simulink model "SoC_modelbased"  (Simulink 10.2)
settings: Solver=ode45  StartTime=0.0  StopTime=75000  RelTol=1e-3  EnableMultiTasking=on
undefined symbols (not defined in the file or in its folder): battery_capacity, capacity_reduction_factor
libraries: pid_lib x1
settings Model: Creator=giovanni  LastModifiedBy=marcomussi
settings DataIOCC: LimitDataPoints=on
settings OptimizationCC: ExpressionDepthLimit=2147483647
settings DebuggingCC: AlgebraicLoopMsg=none  SolverPrmCheckMsg=warning  StateNameClashWarn=warning
settings ConfigComp: CovSFcnEnable=off

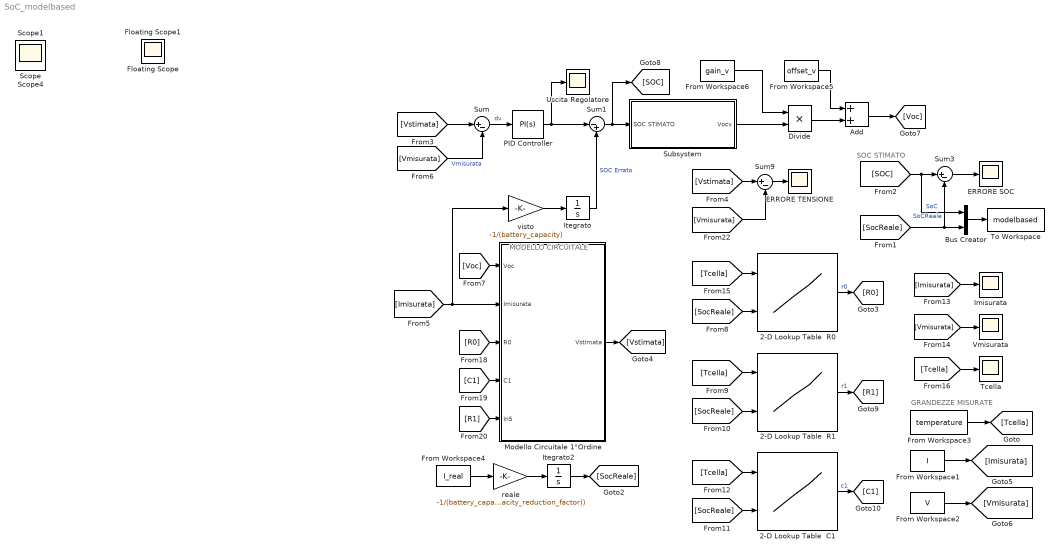
== system SoC_modelbased ==
  note: GRANDEZZE MISURATE
  note: MODELLO CIRCUITALE
  note: SOC STIMATO
  2-D Lookup Table  C1 : Lookup_n-D  BreakpointsForDimension1=[2 10 20 30 40]  BreakpointsForDimension2=|  Table=|  ExtrapMethod=Clip  UseLastTableValue=on  RndMeth=Simplest  InputSameDT=on
      BreakpointsForDimension2=|
      | [0.163145513075157	0.212319317933106	0.261240559284839	0.310166932050155	0.359120506846337	0.408117376969695	0.457142933463410	0.506212254204039	0.555338838203931	0.604575150487779	0.653951958006247	0.703454663475372	0.753095676425974	0.802798623734601	0.852544469586437	0.902318454030865	0.952029425469133
      | ]
      Table=|
      | reshape([4883.03519070804	12169.0591847539	25886.4273045605	38719.3929527266	46611.1569933944	49037.7719780486	48655.0163502780	45651.0467956961	40273.0777451686	37350.2623397049	36077.5767340543	39501.2979937867	41888.5367241290	45944.3440886540	47340.5371368008	40342.5254893418	32279.8355077883
      | ;16734.4447698804	36383.3367558066	10558.5991060525	28700.2818935131	40709.0435359338	41723.5057570253	40864.1569919999	37616.9730750107	35738.8044324206	35170.5298527745	38697.6037402281	40347.5630644685	59786.2011265682	65487.0387899900	52847.2531644424	38384.0954926983	3076.17405677198
      | ;49422.0818325063	44194.6448539184	46689.7389781123	55338.2623186283	57858.9917868986	51557.9597696658	47664.7575534437	45376.1428602184	41998.9090480968	46277.4545844011	63416.5345836845	113830.090748268	87968.0015724581	56812.5882907500	40993.8246669719	33456.6674019576	29472.6682729864
      | ;54635.7828825187	50162.6639997846	53080.5954364735	77121.4914455776	76822.1821718255	64750.1199311789	57640.0479184368	56058.3569816889	55247.8959796781	60526.6599782258	78181.4160334794	84195.4324070183	46800.1200393919	40467.0265124302	41295.1858309488	46698.5369472996	52604.3448750037
      | ;67609.5955014304	62000.5046639622	68058.6226338516	72794.5594133714	96897.9201911745	70944.9748936255	59238.5325083050	60991.2082423147	63036.6077240695	77126.4499717178	84110.6033498963	81077.6225365922	57512.6966769028	47439.9521721272	57512.6966769028	52021.8000128320	56637.9951691813
      | 
      | 
      | ],[5,17])
      settings: InputPortMap=u0,u1
  2-D Lookup Table  R0 : Lookup_n-D  BreakpointsForDimension1=[2 10 20 30 40]  BreakpointsForDimension2=|  Table=|  ExtrapMethod=Clip  UseLastTableValue=on  RndMeth=Simplest  InputSameDT=on
      BreakpointsForDimension2=|
      | [0.163145513075157	0.212319317933106	0.261240559284839	0.310166932050155	0.359120506846337	0.408117376969695	0.457142933463410	0.506212254204039	0.555338838203931	0.604575150487779	0.653951958006247	0.703454663475372	0.753095676425974	0.802798623734601	0.852544469586437	0.902318454030865	0.952029425469133
      | ]
      Table=|
      | reshape([0.00589215125674365	0.00541978470029585	0.00499714093926361	0.00469880416677026	0.00452477438281580	0.00440046739427690	0.00430102180344579	0.00420157621261467	0.00415185341719912	0.00415743483781025	0.00402754642866022	0.00400268503095244	0.00398317110209365	0.00395827628270558	0.00400806592148174	0.00410213062178356	0.00413254001842218
      | ;0.00303709235748072	0.00288392213410238	0.00224119178669128	0.00228298919385116	0.00251100116848569	0.00251100116848569	0.00253586256619347	0.00251431416479960	0.00251100116848569	0.00251100116848569	0.00251100116848569	0.00243641697536235	0.00248941996514812	0.00248941996514812	0.00253586256619348	0.00261389096340554	0.00260819243580551
      | ;0.00174029783954454	0.00166571364642121	0.00161599085100564	0.00154140665788230	0.00154347880206130	0.00151654526017453	0.00151654526017453	0.00151654526017453	0.00146879434389704	0.00146682246475897	0.00146682246475897	0.00144196106705119	0.00146682246475897	0.00146682246475897	0.00149368916328512	0.00149168386246674	0.00149168386246676
      | ;0.00124306988538895	0.00119492158327110	0.00119492158327110	0.00119492158327110	0.00114513318396814	0.00112023898431665	0.00112023898431665	0.00112023898431666	0.00109534478466517	0.00109534478466517	0.00109390149914228	0.00109390149914228	0.00107045058501370	0.00109534478466517	0.00107045058501368	0.00107045058501370	0.00107045058501370
      | ;0.00124306988538895	0.00119492158327110	0.00119492158327110	0.00119492158327110	0.00114513318396814	0.00112023898431665	0.00112023898431665	0.00112023898431666	0.00109534478466517	0.00109534478466517	0.00109390149914228	0.00109390149914228	0.00107045058501370	0.00109534478466517	0.00107045058501368	0.00107045058501370	0.00107045058501370
      | ],[5,17])
      settings: InputPortMap=u0,u1
  2-D Lookup Table  R1 : Lookup_n-D  BreakpointsForDimension1=[2 10 20 30 40]  BreakpointsForDimension2=[0.163145513075157,0.212319317933106,0.261240559284839,0.310166932050155,0.359120506846337,0.408117376969695,0.45714293346341,0.506212254204039,0.555338838203931,0.604575150487779,0.653951958006247,0.703454663475372,0.753095676425974,0.802798623734601,0.852544469586437,0.902318454030865,0.952029425469133]  Table=|  ExtrapMethod=Clip  UseLastTableValue=on  RndMeth=Simplest  InputSameDT=on
      | reshape([0.00502453534827717	0.00367588701990665	0.00319247881265890	0.00302993723332561	0.00291982270900464	0.00285920460919002	0.00278276741846845	0.00264306089997957	0.00243570269276068	0.00216294341188147	0.00203305616129393	0.00202241994653573	0.00209682119046169	0.00221692502044170	0.00230808320822540	0.00228466445960682	0.00209631440768531
      | ;0.00266398817875266	0.00238618270452139	0.00447070124753020	0.00281597061324941	0.00246711975326851	0.00239381727480884	0.00226853192994109	0.00211471233668856	0.00188813752003067	0.00168213406918835	0.00156890065367138	0.00170717737832054	0.00184429212420431	0.00199083406308978	0.00196226143008924	0.00184884042854420	0.00477068036872411
      | ;0.00145489930127803	0.00144401935773684	0.00138575178024073	0.00153689895358668	0.00155566115621615	0.00147125166882435	0.00134912789326834	0.00121745723839334	0.00114384057312595	0.00104682032934108	0.00105635113191740	0.00137995854070415	0.00147714657103215	0.00140642118925139	0.00129159999177379	0.00116013247107786	0.00107699920727854
      | ;0.000892800723516686	0.000900368902969211	0.000825628019922922	0.000894961231413160	0.000974591258870852	0.000892661782685876	0.000805865664234186	0.000734497793356133	0.000690782187561293	0.000654226098238264	0.000714200349863488	0.000962739095749050	0.000920773665929772	0.000801291777456879	0.000703755429644830	0.000612733520111293	0.000542185281425989
      | ;0.000569524815290559	0.000589671691314312	0.000521991024431531	0.000565743321181922	0.000723068922556481	0.000662261851739134	0.000611925261719721	0.000557262981118940	0.000514286700725400	0.000479209702618554	0.000534595587477637	0.000782980546287748	0.000677393622516657	0.000587227029500275	0.000506737341905882	0.000468493224408239	0.000435772475693713
      | 
      | ],[5,17])
      settings: InputPortMap=u0,u1
  Add : Sum
  Bus Creator : BusCreator  Inputs=2
  Divide : Product  Inputs=**
  ERRORE SOC : Scope
  ERRORE TENSIONE : Scope
  From Workspace1 : FromWorkspace  VariableName=I  SampleTime=1
  From Workspace2 : FromWorkspace  VariableName=V  SampleTime=1
  From Workspace3 : FromWorkspace  VariableName=temperature  SampleTime=1
  From Workspace4 : FromWorkspace  VariableName=I_real  SampleTime=1
  From Workspace5 : FromWorkspace  VariableName=offset_v  SampleTime=1
  From Workspace6 : FromWorkspace  VariableName=gain_v  SampleTime=1
  Imisurata : Scope
  Itegrato : Integrator  InitialCondition=0.55
  Itegrato2 : Integrator  InitialCondition=0.55
  Modello Circuitale 1°Ordine : Subsystem
  PID Controller : pid_lib/PID Controller  Controller=PI  Form=Parallel  TimeDomain=Continuous-time  UseExternalTs=off  SampleTime=1  IntegratorMethod=Forward Euler  FilterMethod=Forward Euler  ControllerParametersSource=internal  P=0  I=0.01  D=0  UseFilter=on  N=100  TunerSelectOption=Transfer Function Based (PID Tuner App)  InitialConditionSource=internal  InitialConditionForIntegrator=0  InitialConditionForFilter=0  DifferentiatorICPrevScaledInput=0  ExternalReset=none  TrackingMode=off  Kt=1  LimitOutput=off  SatLimitsSource=internal  UpperSaturationLimit=inf  LowerSaturationLimit=-inf  LinearizeAsGain=off  AntiWindupMode=none  Kb=1  POutMin=[]  POutMax=[]  IOutMin=[]  IOutMax=[]  DOutMin=[]  DOutMax=[]  NOutMin=[]  NOutMax=[]  SumOutMin=[]  SumOutMax=[]  SaturationOutMin=[]  SaturationOutMax=[]  PParamMin=[]  PParamMax=[]  IParamMin=[]  IParamMax=[]  DParamMin=[]  DParamMax=[]  NParamMin=[]  NParamMax=[]  KbParamMin=[]  KbParamMax=[]  KtParamMin=[]  KtParamMax=[]  KbOutMin=[]  KbOutMax=[]  KtOutMin=[]  KtOutMax=[]  IntegratorOutMin=[]  IntegratorOutMax=[]  FilterOutMin=[]  FilterOutMax=[]  SumI1OutMin=[]  SumI1OutMax=[]  SumI2OutMin=[]  SumI2OutMax=[]  SumI3OutMin=[]  SumI3OutMax=[]  SumI4OutMin=[]  SumI4OutMax=[]  SumDOutMin=[]  SumDOutMax=[]  DifferentiatorOutMin=[]  DifferentiatorOutMax=[]  FilterDiffOutCoefMin=[]  FilterDiffOutCoefMax=[]  ReciprocalOutMin=[]  ReciprocalOutMax=[]  SumDenOutMin=[]  SumDenOutMax=[]  SumNumOutMin=[]  SumNumOutMax=[]  DivideOutMin=[]  DivideOutMax=[]  UdiffTsProdOutMin=[]  UdiffTsProdOutMax=[]  NTsProdOutMin=[]  NTsProdOutMax=[]  UintegralTsProdOutMin=[]  UintegralTsProdOutMax=[]  UngainTsProdOutMin=[]  UngainTsProdOutMax=[]  IntegratorContinuousStateAttributes=''  IntegratorStateMustResolveToSignalObject=off  IntegratorRTWStateStorageClass=Auto  FilterContinuousStateAttributes=''  FilterStateMustResolveToSignalObject=off  FilterRTWStateStorageClass=Auto  ParallelPVariant=InternalParameters  IdealPVariant=Disabled  IVariant=InternalParameters  DVariant=Disabled  IntegratorVariant=Continuous  SatVariant=Disabled  AWVariant=Passthrough  PCopyVariant=Disabled  TRVariant=Disabled  FdbkBlocksVariant=Forward  IdealPFdbkVariant=Disabled  SatFdbkVariant=Disabled  DerivativeFilterVariant=Disabled  NVariant=Disabled  NCopyVariant=Disabled_SignalSpec  FilterICVariant=Disabled  IntegratorICVariant=InternalICs  ExternalResetVariant=Disabled  TRSumVariant=Passthrough  SumFdbkVariant=Disabled  SumVariant=Sum_PI  TsampFilterVariant=InternalTs  TsampNgainVariant=Passthrough  TsampIntegralVariant=Passthrough  ExternalSaturationOutDataTypeStr=Inherit: Same as second input
      link override Integral Gain: Gain=I  Multiplication=Element-wise(K.*u)  ParamMin=IParamMin  ParamMax=IParamMax  ParamDataTypeStr=IParamDataTypeStr  OutMin=IOutMin  OutMax=IOutMax  OutDataTypeStr=IOutDataTypeStr  SampleTime=-1
  Subsystem : Subsystem
  Sum : Sum  Inputs=|+-
  Sum1 : Sum  Inputs=|-+
  Sum3 : Sum  Inputs=|+-
  Sum9 : Sum  Inputs=|+-
  Tcella : Scope
  To Workspace : ToWorkspace  VariableName=modelbased  SaveFormat=Timeseries  SampleTime=-1
  Uscita Regolatore : Scope
  Vmisurata : Scope
  reale : Gain  Gain=-1/(battery_capacity*(1-capacity_reduction_factor))
  visto : Gain  Gain=-1/(battery_capacity)
  Floating Scope : Scope
  Floating Scope1 : Scope
  Scope : Scope
  Scope1 : Scope
  Scope4 : Scope
  wires:
  From Workspace1/1 -> [Imisurata]
  From Workspace2/1 -> [Vmisurata]
  [Voc] -> Modello Circuitale 1°Ordine/1(Voc)
  [R1] -> Modello Circuitale 1°Ordine/5(In5)
  [R0] -> Modello Circuitale 1°Ordine/3(R0)
  [C1] -> Modello Circuitale 1°Ordine/4(C1)
  Sum1/1 -> Subsystem/1(SOC STIMATO), [SOC]
  visto/1 -> Itegrato/1
  Itegrato/1 -> Sum1/2  "SOC Errato"
  [Imisurata] -> Modello Circuitale 1°Ordine/2(Imisurata), visto/1
  [SOC] -> Bus Creator/1, Sum3/1  "SoC"
  Sum3/1 -> ERRORE SOC/1
  Modello Circuitale 1°Ordine/1(Vstimata) -> [Vstimata]
  [Imisurata] -> Imisurata/1
  [Vmisurata] -> Vmisurata/1
  [Tcella] -> Tcella/1
  reale/1 -> Itegrato2/1
  From Workspace4/1 -> reale/1
  [SocReale] -> Bus Creator/2, Sum3/2  "SoCReale"
  [Vstimata] -> Sum/1
  [Vmisurata] -> Sum/2  "Vmisurata"
  PID Controller/1 -> Sum1/1, Uscita Regolatore/1
  [Vstimata] -> Sum9/1
  [Vmisurata] -> Sum9/2
  Sum9/1 -> ERRORE TENSIONE/1
  Sum/1 -> PID Controller/1  "dv"
  Itegrato2/1 -> [SocReale]
  Bus Creator/1 -> To Workspace/1
  [SocReale] -> 2-D Lookup Table  R0/2
  2-D Lookup Table  R0/1 -> [R0]  "r0"
  [SocReale] -> 2-D Lookup Table  R1/2
  [Tcella] -> 2-D Lookup Table  R0/1
  2-D Lookup Table  R1/1 -> [R1]  "r1"
  [Tcella] -> 2-D Lookup Table  R1/1
  [Tcella] -> 2-D Lookup Table  C1/1
  2-D Lookup Table  C1/1 -> [C1]  "c1"
  [SocReale] -> 2-D Lookup Table  C1/2
  From Workspace3/1 -> [Tcella]
  From Workspace5/1 -> Add/1
  Divide/1 -> Add/2
  Add/1 -> [Voc]
  From Workspace6/1 -> Divide/1
  Subsystem/1(Vocv) -> Divide/2

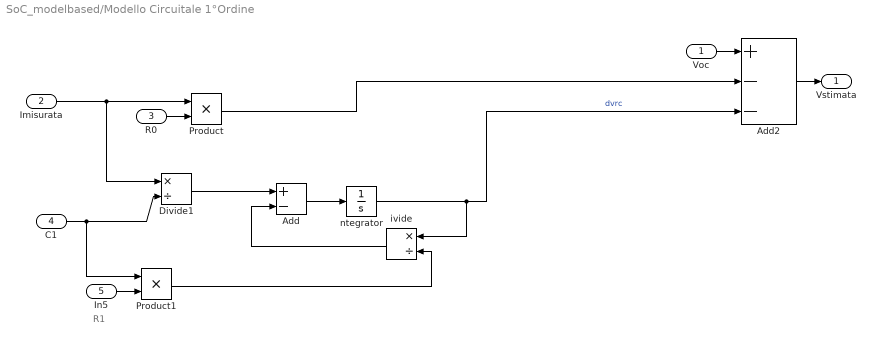
== system SoC_modelbased/Modello Circuitale 1°Ordine ==
  note: R1
  Voc : Inport
  Imisurata : Inport  Port=2
  R0 : Inport  Port=3
  C1 : Inport  Port=4
  In5 : Inport  Port=5
  Add : Sum  Inputs=+-
  Add2 : Sum  Inputs=+--
  Divide1 : Product  Inputs=*/
  Product : Product  RndMeth=Zero
  Product1 : Product  RndMeth=Zero
  ivide : Product  Inputs=*/
  ntegrator : Integrator
  Vstimata : Outport  VectorParamsAs1DForOutWhenUnconnected=off
  wires:
  Product/1 -> Add2/2
  ivide/1 -> Add/2
  Product1/1 -> ivide/2
  Divide1/1 -> Add/1
  C1/1 -> Divide1/2, Product1/1
  ntegrator/1 -> ivide/1, Add2/3  "dvrc"
  Add/1 -> ntegrator/1
  Imisurata/1 -> Product/1, Divide1/1
  Voc/1 -> Add2/1
  Add2/1 -> Vstimata/1
  R0/1 -> Product/2
  In5/1 -> Product1/2

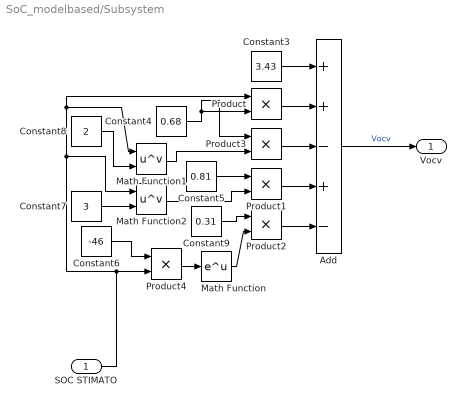
== system SoC_modelbased/Subsystem ==
  SOC STIMATO : Inport
  Add : Sum  Inputs=++-+-
  Constant3 : Constant  Value=3.43
  Constant4 : Constant  Value=0.68
  Constant5 : Constant  Value=0.81
  Constant6 : Constant  Value=-46
  Constant7 : Constant  Value=3
  Constant8 : Constant  Value=2
  Constant9 : Constant  Value=0.31
  Math Function : Math  SaturateOnIntegerOverflow=on
  Math Function1 : Math  Operator=pow  SaturateOnIntegerOverflow=on
  Math Function2 : Math  Operator=pow  SaturateOnIntegerOverflow=on
  Product{,1..4} (5 alike) : Product
  Vocv : Outport
  wires:
  Math Function2/1 -> Product1/2
  Constant6/1 -> Product4/1
  Product3/1 -> Add/3
  Add/1 -> Vocv/1  "Vocv"
  Product2/1 -> Add/5
  Math Function1/1 -> Product3/2
  Math Function/1 -> Product2/2
  Constant8/1 -> Math Function1/2
  Product/1 -> Add/2
  Constant9/1 -> Product2/1
  Constant4/1 -> Product3/1, Product/2
  Product1/1 -> Add/4
  Constant3/1 -> Add/1
  Constant7/1 -> Math Function2/2
  Product4/1 -> Math Function/1
  Constant5/1 -> Product1/1
  SOC STIMATO/1 -> Math Function2/1, Product/1, Math Function1/1, Product4/2
